simulink model "sfcar_vr_observer"  (Simulink 4.00)
settings: Solver=ode5  SolverMode=SingleTasking  StartTime=0.0  StopTime=30  RelTol=1e-3  AbsTol=1e-6
PreLoadFcn:
  | load sf_cardat
undefined symbols (not defined in the file): converter_data, Iei
libraries: simulink3 x3, vrlib x3
settings Model: Creator=nikita  LastModifiedBy=Danek  SaveTime=off  SaveOutput=off  LimitDataPoints=off  IntegerOverflowMsg=none  RTWOptions="-aLogVarNameModifier=\"rt_\" -aExtMode=0 -aRollThreshold=5 -aShowEliminatedStatements=1 -aRTWVerbose=1 -aInlineInvariantSignals=1 -aLocalBlockOutputs=1 -aInlineParameters=0"  ExtModeTrigMode=oneshot  ExtModeArmWhenConnect=off  ExtModeAutoUpdateStatusClock=off  BlockReductionOpt=off

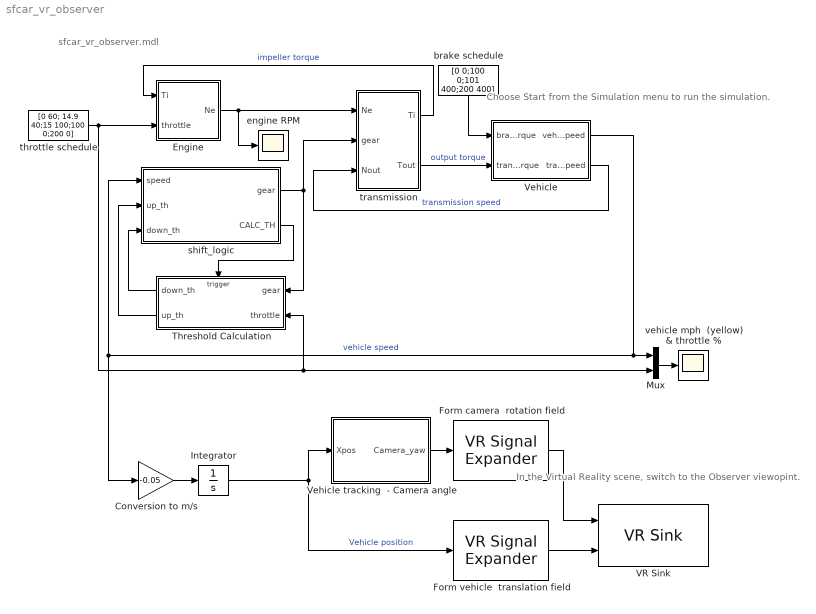
== system sfcar_vr_observer ==
  note: Choose Start from
      | the Simulation menu
      | to run the simulation.
  note: sfcar_vr_observer.mdl
  note: In the Virtual Reality
      |  scene, switch to the
      | Observer viewopint.
  Conversion to m/s : Gain  Gain=-0.05  Multiplication=Element-wise(K.*u)  SaturateOnIntegerOverflow=on
  Engine : Subsystem
      settings: RTWFcnNameOpts=Auto  RTWFileNameOpts=Auto
  Form camera  rotation field : vrlib/VR Signal Expander  outwidth=4  outidx=[4]
  Form vehicle  translation field : vrlib/VR Signal Expander  outwidth=3  outidx=[1]
  Integrator : Integrator  ExternalReset=none  InitialConditionSource=internal  InitialCondition=0  LimitOutput=off  UpperSaturationLimit=inf  LowerSaturationLimit=-inf  ShowSaturationPort=off  ShowStatePort=off  AbsoluteTolerance=auto
  Mux : Mux  Inputs=2
      settings: DisplayOption=none
  Threshold Calculation : Subsystem  Orientation=left  TreatAsAtomicUnit=on
      settings: RTWFcnNameOpts=Auto  RTWFileNameOpts=Auto
  VR Sink : vrlib/VR Sink  SampleTime=0.1  ViewEnable=on  RemoteChange=off  RemoteView=off  FieldsWritten=Camera2.rotation#Octavia.translation  WorldFileName=blossom_skoda.wrl  WorldDescription=Skoda Octavia on UCLA Pearlblossom Highway
  Vehicle : Subsystem  mask(vehicle model){@1=vehicledata(1), @2=vehicledata(2), @3=vehicledata(3), @4=vehicledata(4), @5=vehicledata(5), @6=vehicledata(6)/vehicledata(4)*vehicledata(1)}
      mask prompts: @1 "final drive ratio"; @2 "drag friction at wheels"; @3 "aerodynamic drag"; @4 "wheel radius"; @5 "vehicle inertia"; @6 "initial transmission output speed"
      mask help: vehicle dynamics: torque input from trans., outputs are input speed (transmission output) and vehicle speed
      mask init:
      | Rfd = @1; rload0 = @2; rload2 = @3; Rw = @4; Iv = @5; N20 = @6;
      settings: RTWFcnNameOpts=Auto  RTWFileNameOpts=Auto
      mask Display: plot([cos(pi*[0:5:360]/180) + 6], [sin(pi*[0:5:360]/180) + 1.5],[cos(pi*[0:5:360]/180) + 1], [sin(pi*[0:5:360]/180) + 4], [10 7.5 6.75], [3.5 1 1.5], [10 9.75 7.5 6.25 3 1.5 4 5 7.5], [3.5 4.75 5.5 7 8 7 6 4 5.5], [6.5 4], [7 6], [5.25 2], [2 4], [7.5 1 0], [2.5 6 6.5], [7.5 7.25 9.75], [1 2.25 4.75], [2.75 2 0 0 0.25], [7.5 8 6.5 5.25 5], [1.5 0.5], [6.75 6.25])
  Vehicle tracking  - Camera angle : Subsystem
      settings: RTWFcnNameOpts=Auto  RTWFileNameOpts=Auto
  brake schedule : FromWorkspace  Orientation=down  VariableName=[0 0;100 0;101 400;200 400]  SampleTime=0  OutputAfterFinalValue=Extrapolation
  engine RPM : Scope
      settings: TickLabels=on  TimeRange=auto  YMin=0  YMax=6000  SaveToWorkspace=off  SaveName=ScopeData  DataFormat=Array  LimitDataPoints=on  MaxDataPoints=5000
  shift_logic : Stateflow chart
      settings: RTWFcnNameOpts=Auto  RTWFileNameOpts=Auto
  throttle schedule : FromWorkspace  VariableName=[0 60; 14.9 40;15 100;100 0;200 0]  SampleTime=0  OutputAfterFinalValue=Extrapolation
  transmission : Subsystem
      settings: RTWFcnNameOpts=Auto  RTWFileNameOpts=Auto
  vehicle mph  (yellow) & throttle % : Scope
      settings: TickLabels=on  TimeRange=auto  YMin=0  YMax=140  SaveToWorkspace=off  SaveName=ScopeData  DataFormat=Array  LimitDataPoints=on  MaxDataPoints=5000
  wires:
  brake schedule/1 -> Vehicle/1(brake torque)
  transmission/1(Ti) -> Engine/1(Ti)  "impeller torque"
  throttle schedule/1 -> Engine/2(throttle), Mux/2, Threshold Calculation/2(throttle)
  Engine/1(Ne) -> transmission/1(Ne), engine RPM/1
  transmission/2(Tout) -> Vehicle/2(transmission output torque)  "output torque"
  Vehicle/2(transmission output speed) -> transmission/3(Nout)  "transmission speed"
  Threshold Calculation/1(down_th) -> shift_logic/3(down_th)
  Threshold Calculation/2(up_th) -> shift_logic/2(up_th)
  shift_logic/1(gear) -> transmission/2(gear), Threshold Calculation/1(gear)
  shift_logic/2(CALC_TH) -> Threshold Calculation/Trigger
  Vehicle/1(vehicle speed) -> Mux/1, shift_logic/1(speed), Conversion to m/s/1  "vehicle speed"
  Mux/1 -> vehicle mph  (yellow) & throttle %/1
  Conversion to m/s/1 -> Integrator/1
  Form vehicle  translation field/1 -> VR Sink/2
  Vehicle tracking  - Camera angle/1(Camera_yaw) -> Form camera  rotation field/1
  Form camera  rotation field/1 -> VR Sink/1
  Integrator/1 -> Vehicle tracking  - Camera angle/1(Xpos), Form vehicle  translation field/1  "Vehicle position"

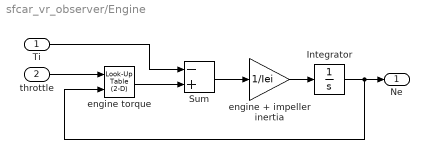
== system sfcar_vr_observer/Engine ==
  Ti : Inport  Port=1  LatchInput=off
  throttle : Inport  Port=2  LatchInput=off
  Integrator : Integrator  ExternalReset=none  InitialConditionSource=internal  InitialCondition=1000  LimitOutput=on  UpperSaturationLimit=6000  LowerSaturationLimit=600  ShowSaturationPort=off  ShowStatePort=off  AbsoluteTolerance=auto
  Sum : Sum  Inputs=-+  SaturateOnIntegerOverflow=on
  engine torque : simulink3/Functions & Tables/Look-Up Table (2-D)  x=thvec  y=nevec  t=emap
  engine + impeller inertia : Gain  Gain=1/Iei  Multiplication=Element-wise(K.*u)  SaturateOnIntegerOverflow=on
  Ne : Outport  Port=1  InitialOutput=0
  wires:
  Ti/1 -> Sum/1
  throttle/1 -> engine torque/1
  Integrator/1 -> engine torque/2, Ne/1
  Sum/1 -> engine + impeller inertia/1
  engine + impeller inertia/1 -> Integrator/1
  engine torque/1 -> Sum/2

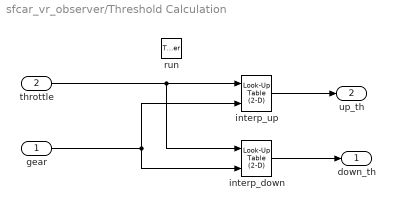
== system sfcar_vr_observer/Threshold Calculation ==
  gear : Inport  Port=1  LatchInput=off
  throttle : Inport  Port=2  LatchInput=off
  run : TriggerPort  TriggerType=function-call  OutputDataType=auto
  interp_down : simulink3/Functions & Tables/Look-Up Table (2-D)  x=downth  y=[1:4]  t=downtab
  interp_up : simulink3/Functions & Tables/Look-Up Table (2-D)  x=upth  y=[1:4]  t=uptab
  down_th : Outport  Port=1
  up_th : Outport  Port=2
  wires:
  interp_up/1 -> up_th/1
  interp_down/1 -> down_th/1
  throttle/1 -> interp_up/1, interp_down/1
  gear/1 -> interp_up/2, interp_down/2

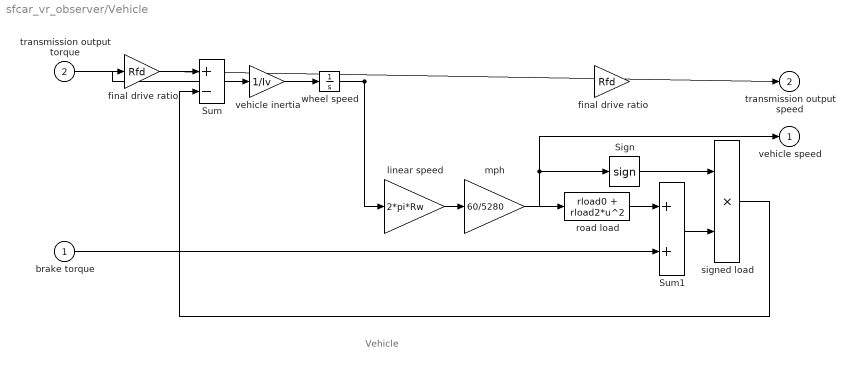
== system sfcar_vr_observer/Vehicle ==
  note: Vehicle
  brake torque : Inport  Port=1  LatchInput=off
  transmission output torque : Inport  Port=2  LatchInput=off
  Sign : Signum
  Sum : Sum  Inputs=+-  SaturateOnIntegerOverflow=on
  Sum1 : Sum  Inputs=++  SaturateOnIntegerOverflow=on
  final drive ratio : Gain  Gain=Rfd  Multiplication=Element-wise(K.*u)  SaturateOnIntegerOverflow=on
  final drive ratio : Gain  Gain=Rfd  Multiplication=Element-wise(K.*u)  SaturateOnIntegerOverflow=on
  linear speed : Gain  Gain=2*pi*Rw  Multiplication=Element-wise(K.*u)  SaturateOnIntegerOverflow=on
  mph : Gain  Gain=60/5280  Multiplication=Element-wise(K.*u)  SaturateOnIntegerOverflow=on
  road load : Fcn  Expr=rload0 + rload2*u^2
  signed load : Product  Inputs=2  Multiplication=Element-wise(.*)  SaturateOnIntegerOverflow=on
  vehicle inertia : Gain  Gain=1/Iv  Multiplication=Element-wise(K.*u)  SaturateOnIntegerOverflow=on
  wheel speed : Integrator  ExternalReset=none  InitialConditionSource=internal  InitialCondition=N20/Rfd  LimitOutput=off  UpperSaturationLimit=inf  LowerSaturationLimit=-inf  ShowSaturationPort=off  ShowStatePort=off  AbsoluteTolerance=auto
  vehicle speed : Outport  Port=1  InitialOutput=0
  transmission output speed : Outport  Port=2  InitialOutput=0
  wires:
  final drive ratio/1 -> transmission output speed/1
  brake torque/1 -> Sum1/2
  Sum1/1 -> signed load/2
  road load/1 -> Sum1/1
  Sign/1 -> signed load/1
  signed load/1 -> Sum/2
  transmission output torque/1 -> final drive ratio/1
  vehicle inertia/1 -> wheel speed/1
  Sum/1 -> vehicle inertia/1
  mph/1 -> vehicle speed/1, Sign/1, road load/1
  linear speed/1 -> mph/1
  wheel speed/1 -> linear speed/1, final drive ratio/1
  final drive ratio/1 -> Sum/1

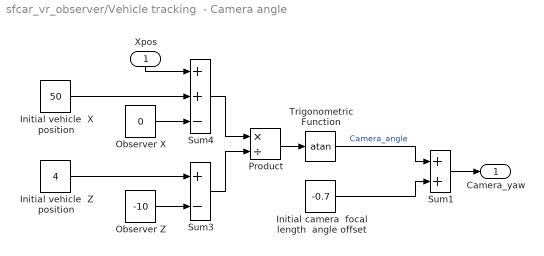
== system sfcar_vr_observer/Vehicle tracking  - Camera angle ==
  Xpos : Inport  Orientation=down  Port=1  LatchInput=off
  Initial camera  focal length  angle offset : Constant  Value=-0.7
  Initial vehicle  X position : Constant  Value=50
  Initial vehicle  Z position : Constant  Value=4
  Observer X : Constant  Value=0
  Observer Z : Constant  Value=-10
  Product : Product  Inputs=*/  Multiplication=Element-wise(.*)  SaturateOnIntegerOverflow=on
  Sum1 : Sum  Inputs=++  SaturateOnIntegerOverflow=on
  Sum3 : Sum  Inputs=+-  SaturateOnIntegerOverflow=on
  Sum4 : Sum  Inputs=++-  SaturateOnIntegerOverflow=on
  Trigonometric Function : Trigonometry  Operator=atan  OutputSignalType=real
  Camera_yaw : Outport  Port=1
  wires:
  Observer Z/1 -> Sum3/2
  Sum3/1 -> Product/2
  Product/1 -> Trigonometric Function/1
  Sum4/1 -> Product/1
  Observer X/1 -> Sum4/3
  Initial vehicle  X position/1 -> Sum4/2
  Initial camera  focal length  angle offset/1 -> Sum1/2
  Trigonometric Function/1 -> Sum1/1  "Camera_angle"
  Sum1/1 -> Camera_yaw/1
  Xpos/1 -> Sum4/1
  Initial vehicle  Z position/1 -> Sum3/1

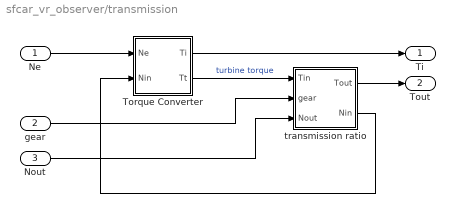
== system sfcar_vr_observer/transmission ==
  Ne : Inport  Port=1  LatchInput=off
  gear : Inport  Port=2  LatchInput=off
  Nout : Inport  Port=3  LatchInput=off
  Torque Converter : Subsystem  mask(torque converter){speedratio=converter_data(:,1), Kfactor=converter_data(:,2), Torkratio=converter_data(:,3)}
      mask prompts: speedratio "speed ratio"; Kfactor "K factor"; Torkratio "torque ratio"
      mask help: torque converter
      settings: RTWFcnNameOpts=Auto  RTWFileNameOpts=Auto
      mask Help: Torque converter input and output torques are computed as a function of the input and output speeds
      mask Display: plot([cos([90:10:450]*pi/180),.63*cos([90:10:450]*pi/180),.63*cos([90:10:240]*pi/180),cos([240:10:300]*pi/180),.63*cos([300]*pi/180)],[sin([90:10:450]*pi/180),.63*sin([90:10:450]*pi/180)+.1,.63*sin([90:10:240]*pi/180)+.1,sin([240:10:300]*pi/180),.63*sin([300]*pi/180)+.1])
  transmission ratio : Subsystem
      settings: RTWFcnNameOpts=Auto  RTWFileNameOpts=Auto
  Ti : Outport  Port=1  InitialOutput=0
  Tout : Outport  Port=2  InitialOutput=0
  wires:
  transmission ratio/1(Tout) -> Tout/1
  Torque Converter/1(Ti) -> Ti/1
  Nout/1 -> transmission ratio/3(Nout)
  gear/1 -> transmission ratio/2(gear)
  Ne/1 -> Torque Converter/1(Ne)
  transmission ratio/2(Nin) -> Torque Converter/2(Nin)
  Torque Converter/2(Tt) -> transmission ratio/1(Tin)  "turbine torque"

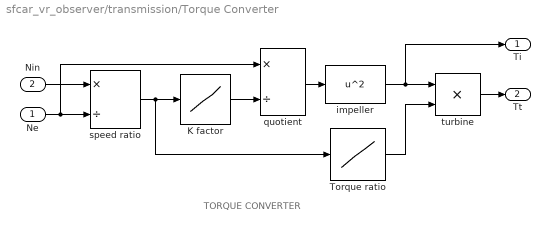
== system sfcar_vr_observer/transmission/Torque Converter ==
  note: TORQUE CONVERTER
  Ne : Inport  Port=1  LatchInput=off
  Nin : Inport  Port=2  LatchInput=off
  K factor : Lookup  InputValues=speedratio  OutputValues=Kfactor
  Torque ratio : Lookup  InputValues=speedratio  OutputValues=Torkratio
  impeller : Fcn  Expr=u^2
  quotient : Product  Inputs=*/  Multiplication=Element-wise(.*)  SaturateOnIntegerOverflow=on
  speed ratio : Product  Inputs=*/  Multiplication=Element-wise(.*)  SaturateOnIntegerOverflow=on
  turbine : Product  Inputs=2  Multiplication=Element-wise(.*)  SaturateOnIntegerOverflow=on
  Ti : Outport  Port=1  InitialOutput=0
  Tt : Outport  Port=2  InitialOutput=0
  wires:
  Torque ratio/1 -> turbine/2
  quotient/1 -> impeller/1
  K factor/1 -> quotient/2
  speed ratio/1 -> Torque ratio/1, K factor/1
  impeller/1 -> turbine/1, Ti/1
  turbine/1 -> Tt/1
  Ne/1 -> speed ratio/2, quotient/1
  Nin/1 -> speed ratio/1

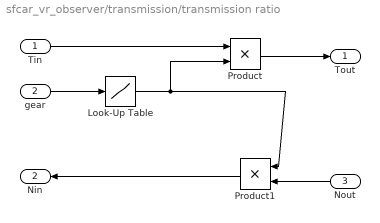
== system sfcar_vr_observer/transmission/transmission ratio ==
  Tin : Inport  Port=1  LatchInput=off
  gear : Inport  Port=2  LatchInput=off
  Nout : Inport  Orientation=left  Port=3  LatchInput=off
  Look-Up Table : Lookup  InputValues=[1 2 3 4]  OutputValues=[2.393 1.450 1.000 0.677]
  Product : Product  Inputs=2  Multiplication=Element-wise(.*)  SaturateOnIntegerOverflow=on
  Product1 : Product  Orientation=left  Inputs=2  Multiplication=Element-wise(.*)  SaturateOnIntegerOverflow=on
  Tout : Outport  Port=1  InitialOutput=0
  Nin : Outport  Orientation=left  Port=2  InitialOutput=0
  wires:
  Look-Up Table/1 -> Product1/1, Product/2
  Nout/1 -> Product1/2
  Product1/1 -> Nin/1
  Product/1 -> Tout/1
  Tin/1 -> Product/1
  gear/1 -> Look-Up Table/1

== stateflow chart shift_logic ==
  settings: updateMethod=DISCRETE  sampleTime=0.04
  state gear_state [parallel]
    state fourth
      entry: gear = 4;
    state second
      entry: gear = 2;
    state third
      entry: gear = 3;
    state first
      entry: gear = 1;
    third -> fourth : UP
    second -> third : UP
    first -> second : UP
    (default) -> first
    fourth -> third : DOWN
    third -> second : DOWN
    second -> first : DOWN
  state selection_state [parallel]
    during: CALC_TH;
    state downshifting
    state upshifting
    state steady_state
    (default) -> steady_state
    steady_state -> upshifting : [speed > up_th]
    steady_state -> downshifting : [speed < down_th]
    upshifting -> steady_state : [speed < up_th]
    downshifting -> steady_state : [speed > down_th]
    downshifting -> steady_state : after(TWAIT,tick)
        | [speed <= down_th]
        | {gear_state.DOWN}
    upshifting -> steady_state : after(TWAIT,tick)
        | [speed >= up_th]
        | {gear_state.UP}
  data: speed input double; gear output uint8 [1..4]; TWAIT constant uint8; up_th input double; down_th input double
  data speed settings: units=double
  data gear settings: units=int
  events: DOWN local EITHER_EDGE_EVENT; UP local EITHER_EDGE_EVENT; CALC_TH output FUNCTION_CALL_EVENT
